simulink model "motorSpeed"  (R2019b)
settings: Solver=VariableStepAuto  StartTime=0.0  StopTime=1  RelTol=1e-3
values from neighbouring files (symbols this model uses):
  b = 0.1    [motorParam.m]
  J = 0.01    [motorParam.m]
  Ke = 0.01    [motorParam.m]
  Kt = 0.01    [motorParam.m]
  L = 0.5    [motorParam.m]
  R = 1    [motorParam.m]
settings Model: Creator=zhaoyuan_huo  LastModifiedBy=zhaoyuan_huo

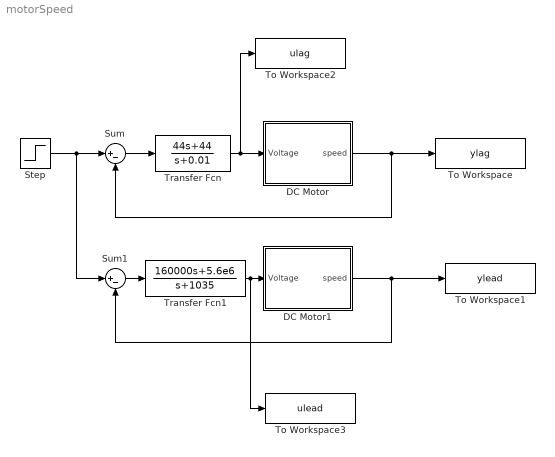
== system motorSpeed ==
  DC Motor : Subsystem
  DC Motor1 : Subsystem
  Step : Step  Time=0  SampleTime=0
  Sum : Sum  Inputs=|+-
  Sum1 : Sum  Inputs=|+-
  To Workspace : ToWorkspace  VariableName=ylag  SampleTime=-1
      settings: Save2DSignal=2-D array (concatenate along first dimension)
  To Workspace1 : ToWorkspace  VariableName=ylead  SampleTime=-1
      settings: Save2DSignal=2-D array (concatenate along first dimension)
  To Workspace2 : ToWorkspace  VariableName=ulag  SampleTime=-1
      settings: Save2DSignal=2-D array (concatenate along first dimension)
  To Workspace3 : ToWorkspace  VariableName=ulead  SampleTime=-1
      settings: Save2DSignal=2-D array (concatenate along first dimension)
  Transfer Fcn : TransferFcn  Numerator=[44 44]  Denominator=[1 0.01]
  Transfer Fcn1 : TransferFcn  Numerator=[160000 5.6e6]  Denominator=[1 1035]
  wires:
  DC Motor/1(speed) -> To Workspace/1, Sum/2
  Sum/1 -> Transfer Fcn/1
  Transfer Fcn/1 -> To Workspace2/1, DC Motor/1(Voltage)
  DC Motor1/1(speed) -> To Workspace1/1, Sum1/2
  Sum1/1 -> Transfer Fcn1/1
  Transfer Fcn1/1 -> To Workspace3/1, DC Motor1/1(Voltage)
  Step/1 -> Sum1/1, Sum/1

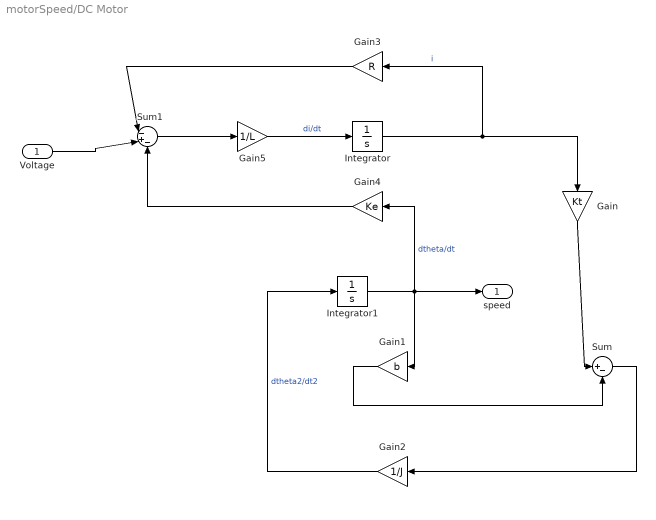
== system motorSpeed/DC Motor ==
  Voltage : Inport
  Gain : Gain  Gain=Kt
  Gain1 : Gain  Gain=b
  Gain2 : Gain  Gain=1/J
  Gain3 : Gain  Gain=R
  Gain4 : Gain  Gain=Ke
  Gain5 : Gain  Gain=1/L
  Integrator : Integrator
  Integrator1 : Integrator
  Sum : Sum  Inputs=|+-
  Sum1 : Sum  Inputs=|-+-
  speed : Outport
  wires:
  Sum1/1 -> Gain5/1
  Gain1/1 -> Sum/2
  Gain5/1 -> Integrator/1  "di/dt"
  Sum/1 -> Gain2/1
  Gain2/1 -> Integrator1/1  "dtheta2/dt2"
  Gain3/1 -> Sum1/1
  Gain4/1 -> Sum1/3
  Integrator/1 -> Gain3/1, Gain/1  "i"
  Gain/1 -> Sum/1
  Voltage/1 -> Sum1/2
  Integrator1/1 -> speed/1, Gain1/1, Gain4/1  "dtheta/dt"

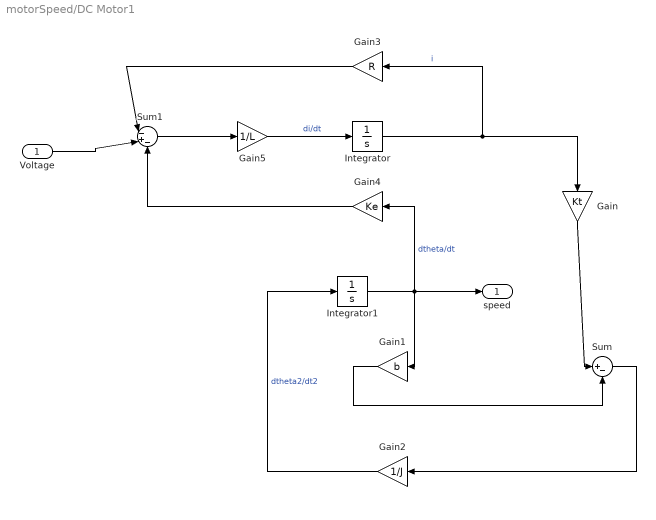
== system motorSpeed/DC Motor1 ==
  Voltage : Inport
  Gain : Gain  Gain=Kt
  Gain1 : Gain  Gain=b
  Gain2 : Gain  Gain=1/J
  Gain3 : Gain  Gain=R
  Gain4 : Gain  Gain=Ke
  Gain5 : Gain  Gain=1/L
  Integrator : Integrator
  Integrator1 : Integrator
  Sum : Sum  Inputs=|+-
  Sum1 : Sum  Inputs=|-+-
  speed : Outport
  wires:
  Sum1/1 -> Gain5/1
  Gain1/1 -> Sum/2
  Gain5/1 -> Integrator/1  "di/dt"
  Sum/1 -> Gain2/1
  Gain2/1 -> Integrator1/1  "dtheta2/dt2"
  Gain3/1 -> Sum1/1
  Gain4/1 -> Sum1/3
  Integrator/1 -> Gain3/1, Gain/1  "i"
  Gain/1 -> Sum/1
  Voltage/1 -> Sum1/2
  Integrator1/1 -> speed/1, Gain1/1, Gain4/1  "dtheta/dt"
